simulink model "test_three_phase_thyristor_rectifier"  (R2018b)
settings: Solver=ode8  StartTime=0.0  StopTime=0.02  FixedStep=1e-6  MaxStep=1e-4  RelTol=1e-3
libraries: powerlib x8, typhoonHILlib x1
settings Model: Creator=Marcos  LastModifiedBy=USER
settings SFSimCC: SimUseLocalCustomCode=off
settings RTWCC: RTWUseLocalCustomCode=off

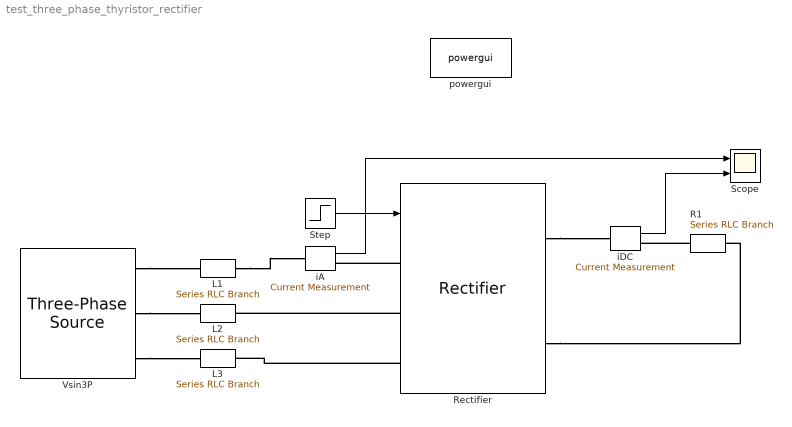
== system test_three_phase_thyristor_rectifier ==
  L1 : powerlib/Elements/Series RLC Branch  LConnTagsString=__new0  RConnTagsString=__new0  BranchType=L  Resistance=10  Inductance=10e-6  SetiL0=off  InitialCurrent=0  Capacitance=1e-6  Setx0=off  InitialVoltage=0  Measurements=None
      settings: SourceProductName=Simscape Electrical
  L2 : powerlib/Elements/Series RLC Branch  LConnTagsString=__new0  RConnTagsString=__new0  BranchType=L  Resistance=10  Inductance=10e-6  SetiL0=off  InitialCurrent=0  Capacitance=1e-6  Setx0=off  InitialVoltage=0  Measurements=None
      settings: SourceProductName=Simscape Electrical
  L3 : powerlib/Elements/Series RLC Branch  LConnTagsString=__new0  RConnTagsString=__new0  BranchType=L  Resistance=10  Inductance=10e-6  SetiL0=off  InitialCurrent=0  Capacitance=1e-6  Setx0=off  InitialVoltage=0  Measurements=None
      settings: SourceProductName=Simscape Electrical
  R1 : powerlib/Elements/Series RLC Branch  LConnTagsString=__new0  RConnTagsString=__new0  BranchType=R  Resistance=10  Inductance=1e-3  SetiL0=off  InitialCurrent=0  Capacitance=1e-6  Setx0=off  InitialVoltage=0  Measurements=None
      settings: SourceProductName=Simscape Electrical
  Rectifier : typhoonHILlib/Rectifier  RecType=Thyristor  ThreePhase=on  sa_top_logic=Active-high  sa_bot_logic=Active-high  sb_top_logic=Active-high  sb_bot_logic=Active-high  sc_top_logic=Active-high  sc_bot_logic=Active-high  di_sa_top=1  di_sa_bot=2  di_sb_top=3  di_sb_bot=4  di_sc_top=5  di_sc_bot=6  v_sa_top=off  i_sa_top=off  v_sa_bot=off  i_sa_bot=off  v_sb_top=off  i_sb_top=off  v_sb_bot=off  i_sb_bot=off  v_sc_top=off  i_sc_top=off  v_sc_bot=off  i_sc_bot=off  r_on=0.001  v_f=0  r_s=1e5  c_s=inf  toggle_init=on  toggle_draw=on  model_loaded=off  old_pat=typhoonPatterns/Thyristor Rectifier (3-Phase)  old_size=145,210
      settings: SourceProductName=Typhoon HIL
  Scope : Scope  NumInputPorts=2
  Step : Step  Time=0.005  Before=[0 0 0 0 0 0]  After=[1 1 1 1 1 1]  SampleTime=0
  Vsin3P : powerlib/Electrical Sources/Three-Phase Source  InternalConnection=Yg  VoltagePhases=off  Voltage=381  PhaseAngle=0  Voltage_phases=[25e3 25e3 25e3]/sqrt(3)  PhaseAngles_phases=[0 -120 +120]  Frequency=50  NonIdealSource=off  SpecifyImpedance=off  Resistance=0.8929  Inductance=16.58e-3  ShortCircuitLevel=100e6  BaseVoltage=25e3  XRratio=7  BusType=swing  Pref=10e3  Qref=0  Prefabc=[10e3, 10e3, 10e3]  Qrefabc=[0, 0, 0]  Qmin=-inf  Qmax=inf
      settings: SourceProductName=Simscape Electrical
  iA : powerlib/Measurements/Current Measurement  PhasorSimulation=off  OutputType=Complex  PSBequivalent=0
      settings: SourceProductName=Simscape Electrical
  iDC : powerlib/Measurements/Current Measurement  PhasorSimulation=off  OutputType=Complex  PSBequivalent=0
      settings: SourceProductName=Simscape Electrical
  powergui : powerlib/powergui  Priority=1  SimulationMode=Discrete  SampleTime=1e-6  frequency=60  Iterations=50  frequencyindice=50  Pbase=100e6  ErrMax=1e-4  UnitsV=kV  UnitsW=MW  buscounter=0  FunctionMessages=off  echomessages=off  EnableUseOfTLC=off  CurrentSourceSwitches=off  DisableSnubberDevices=off  DisableRonSwitches=off  DisableVfSwitches=off  DisplayEquations=off  SolverType=Tustin/Backward Euler (TBE)  Interpol=off  ExternalGateDelay=off  methode=off  Ts=100  x0status=blocks  SPID=on  SwTol=0  HookPort=off  RestoreLinks=warning  ResistiveCurrentMeasurement=off  Frange=[0:2:500]  Ylog=off  Xlog=on  ShowGrid=off  save=off  variable=ZData  structure=0  ZoomFFT=off  StartTime=0.0  cycles=1  DisplayStyle=1  fundamental=60  FreqAxis=off  MaxFrequency=1000  frequencyindicesteady=1  RmsSteady=1  display=off
      settings: SourceProductName=Simscape Electrical
  wires:
  Step/1 -> Rectifier/1
  iDC/1 -> Scope/2
  iA/1 -> Scope/1
  connections:
  R1/LConn1 -- iDC/RConn1
  Rectifier/RConn1 -- iDC/LConn1
  Rectifier/RConn2 -- R1/RConn1
  Rectifier/LConn1 -- iA/RConn1
  Rectifier/LConn2 -- L2/RConn1
  Vsin3P/RConn3 -- L3/LConn1
  L1/RConn1 -- iA/LConn1
  Vsin3P/RConn1 -- L1/LConn1
  Vsin3P/RConn2 -- L2/LConn1
  Rectifier/LConn3 -- L3/RConn1
